simulink model "Question1"  (R2025a)
settings: Solver=VariableStepAuto  StartTime=0.0  StopTime=5  RelTol=1e-3
values from neighbouring files (symbols this model uses):
  ax = -5    [evasion.m]
  d = 3.5    [evasion.m]
  g = 9.81    [evasion.m]
  mu = 0.85    [evasion.m]
libraries: SignalEditorBlockLib x2
settings Model: Creator=mefat  LastModifiedBy=mefat

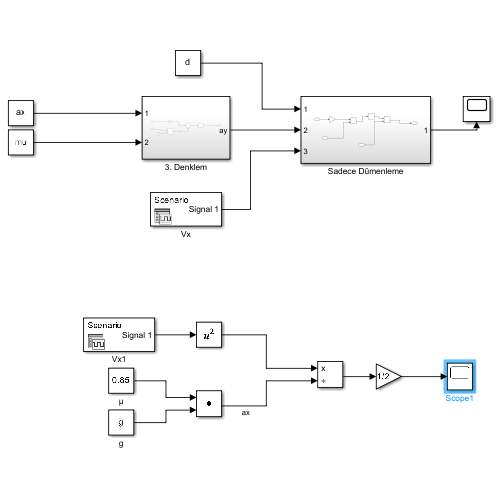
[thumbnail: Simulink's stored preview of the top-level diagram]
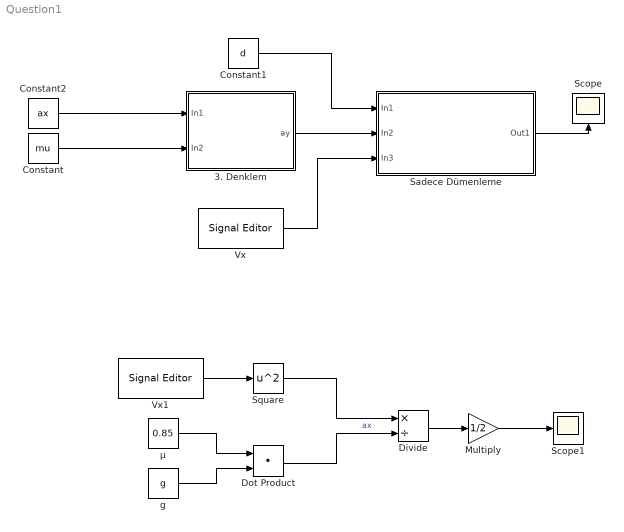
== system Question1 ==
  3. Denklem : Subsystem
  Constant : Constant  Value=mu
  Constant1 : Constant  Value=d
  Constant2 : Constant  Value=ax
  Divide : Product  Inputs=*/
  Dot Product : DotProduct  OutDataTypeStr=Inherit: Inherit via internal rule
  Multiply : Gain  Gain=1/2
  Sadece Dümenleme : Subsystem
  Scope : Scope
      settings: ActiveDisplayYMinimum=-8.0050372802259488  ActiveDisplayYMaximum=77.719593000904254
  Scope1 : Scope
      settings: ActiveDisplayYMinimum=-26.546041454298319  ActiveDisplayYMaximum=238.914373088685
  Square : Math  Operator=square
  Vx : SignalEditorBlockLib/Signal Editor  FileName=untitled.mat  ActiveScenario=Scenario  ActiveSignal=Signal 1  IsBus=off  OutputBusObjectStr=Bus: BusObject  SampleTime=0  ZeroCross=off  OutputAfterFinalValue=Setting to zero  Unit=inherit  PreserveSignalName=on  ApplySigPropsToAllScenarios=on  ApplySigPropsToAllSignals=off  SignalPropertySource=Dialog parameters
  Vx1 : SignalEditorBlockLib/Signal Editor  FileName=untitled.mat  ActiveScenario=Scenario  ActiveSignal=Signal 1  IsBus=off  OutputBusObjectStr=Bus: BusObject  SampleTime=0  ZeroCross=off  OutputAfterFinalValue=Setting to zero  Unit=inherit  PreserveSignalName=on  ApplySigPropsToAllScenarios=on  ApplySigPropsToAllSignals=off  SignalPropertySource=Dialog parameters
  g : Constant  Value=g
  μ : Constant  Value=0.85
  wires:
  Constant2/1 -> 3. Denklem/1(In1)
  Constant/1 -> 3. Denklem/2(In2)
  Constant1/1 -> Sadece Dümenleme/1(In1)
  3. Denklem/1(ay) -> Sadece Dümenleme/2(In2)
  Vx/1 -> Sadece Dümenleme/3(In3)
  Sadece Dümenleme/1(Out1) -> Scope/1
  μ/1 -> Dot Product/1
  g/1 -> Dot Product/2
  Dot Product/1 -> Divide/2  "ax"
  Vx1/1 -> Square/1
  Square/1 -> Divide/1
  Divide/1 -> Multiply/1
  Multiply/1 -> Scope1/1

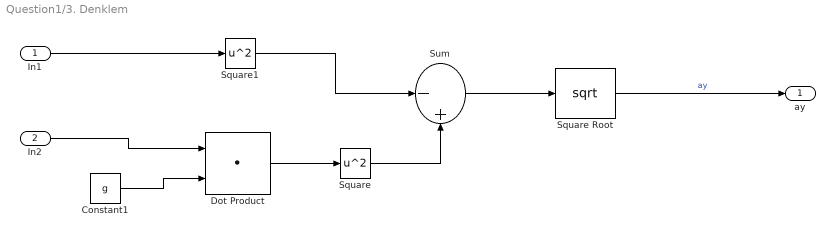
== system Question1/3. Denklem ==
  In1 : Inport
  In2 : Inport  Port=2
  Constant1 : Constant  Value=g
  Dot Product : DotProduct  OutDataTypeStr=Inherit: Inherit via internal rule
  Square : Math  Operator=square
  Square Root : Sqrt
  Square1 : Math  Operator=square
  Sum : Sum  Inputs=|-+
  ay : Outport
  wires:
  Constant1/1 -> Dot Product/2
  In2/1 -> Dot Product/1
  Dot Product/1 -> Square/1
  Sum/1 -> Square Root/1
  In1/1 -> Square1/1
  Square Root/1 -> ay/1  "ay"
  Square1/1 -> Sum/1
  Square/1 -> Sum/2

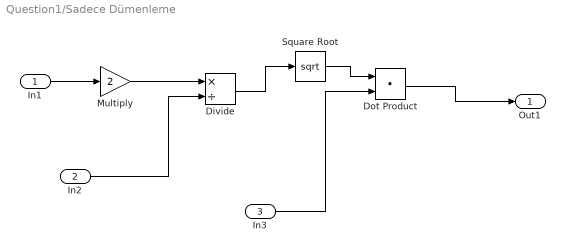
== system Question1/Sadece Dümenleme ==
  In1 : Inport
  In2 : Inport  Port=2
  In3 : Inport  Port=3
  Divide : Product  Inputs=*/
  Dot Product : DotProduct  OutDataTypeStr=Inherit: Inherit via internal rule
  Multiply : Gain  Gain=2
  Square Root : Sqrt
  Out1 : Outport
  wires:
  In2/1 -> Divide/2
  Multiply/1 -> Divide/1
  Square Root/1 -> Dot Product/1
  In3/1 -> Dot Product/2
  Dot Product/1 -> Out1/1
  Divide/1 -> Square Root/1
  In1/1 -> Multiply/1
